simulink model "RM_NSMC"  (R2018b)
settings: Solver=VariableStepAuto  StartTime=0.0  StopTime=100  RelTol=1e-3  EnableMultiTasking=on
settings Model: Creator=Administrator  LastModifiedBy=chengqian
settings OptimizationCC: LifeSpan=inf
settings DebuggingCC: LibraryContextMissingDiagnostic=none  SFUnexpectedBacktrackingDiag=warning  SFNoUnconditionalDefaultTransitionDiag=warning  SFExecutionAtInitializationDiag=none
settings SFSimCC: SimUseLocalCustomCode=off
settings RTWCC: RTWUseLocalCustomCode=off
settings CodeAppCC: StateflowObjectComments=on
settings GRTTargetCC: TargetLangStandard=C89/C90 (ANSI)  GeneratePreprocessorConditionals=Disable all
settings ConfigComp: CovMetricSettings=dw  CovHtmlReporting=on  CovSaveCumulativeToWorkspaceVar=on  CovSaveSingleToWorkspaceVar=on  CovExternalEMLEnable=off

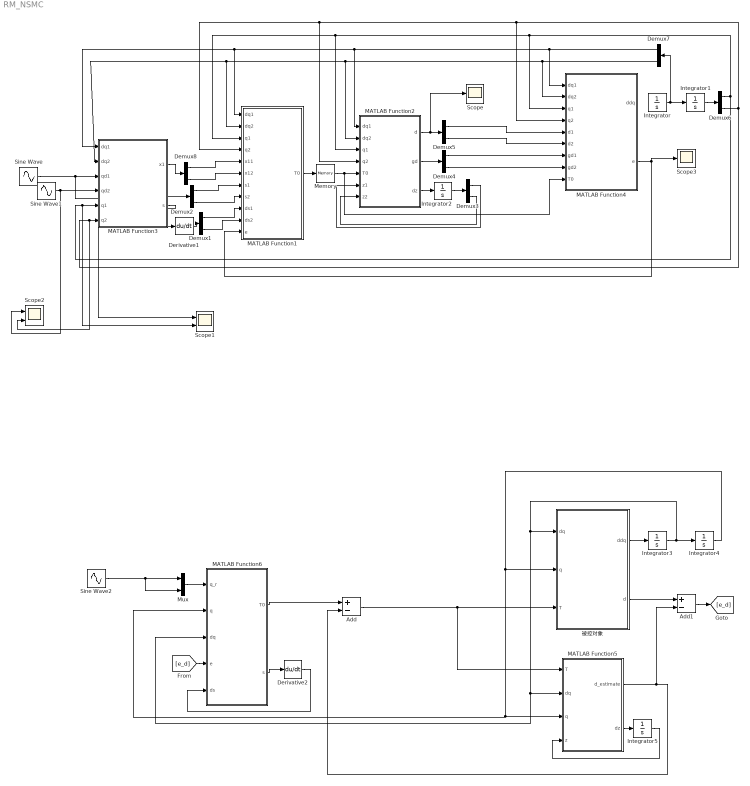
== system RM_NSMC ==
  Add : Sum  Inputs=+-
  Add1 : Sum  Inputs=+-
  Demux{1..8} (8 alike) : Demux  Outputs=2
  Derivative1 : Derivative
  Derivative2 : Derivative
  Integrator{,1..5} (6 alike) : Integrator
  MATLAB Function1 : MATLAB Function  TreatAsAtomicUnit=on
  MATLAB Function2 : MATLAB Function  TreatAsAtomicUnit=on
  MATLAB Function3 : MATLAB Function  TreatAsAtomicUnit=on
  MATLAB Function4 : MATLAB Function  TreatAsAtomicUnit=on
  MATLAB Function5 : MATLAB Function  TreatAsAtomicUnit=on
  MATLAB Function6 : MATLAB Function  TreatAsAtomicUnit=on
  Memory : Memory
  Mux : Mux  Inputs=2
  Scope : Scope
  Scope1 : Scope  NumInputPorts=2
  Scope2 : Scope  NumInputPorts=2
  Scope3 : Scope
  Sine Wave : Sin  SampleTime=0
  Sine Wave1 : Sin  SampleTime=0
  Sine Wave2 : Sin  SampleTime=0
  被控对象 : MATLAB Function  TreatAsAtomicUnit=on
  wires:
  Sine Wave1/1 -> Scope2/1, MATLAB Function3/4(qd2)
  Sine Wave/1 -> Scope1/1, MATLAB Function3/3(qd1)
  ? -> Integrator/1
  Integrator/1 -> Integrator1/1, Demux7/1
  MATLAB Function2/3(dz) -> Integrator2/1
  MATLAB Function3/1(x1) -> Demux8/1
  MATLAB Function3/2(s) -> Derivative1/1, Demux2/1
  Derivative1/1 -> Demux1/1
  Demux1/1 -> MATLAB Function1/9(ds1)
  Demux1/2 -> MATLAB Function1/10(ds2)
  Demux2/1 -> MATLAB Function1/7(s1)
  Demux2/2 -> MATLAB Function1/8(s2)
  Integrator2/1 -> Demux3/1
  Demux3/1 -> MATLAB Function2/6(z1)
  Demux3/2 -> MATLAB Function2/7(z2)
  MATLAB Function2/2(gd) -> Demux4/1
  Demux4/1 -> MATLAB Function4/7(gd1)
  Demux4/2 -> MATLAB Function4/8(gd2)
  MATLAB Function2/1(d) -> Scope/1, Demux5/1
  Demux5/1 -> MATLAB Function4/5(d1)
  Demux5/2 -> MATLAB Function4/6(d2)
  Integrator1/1 -> Demux6/1
  Demux6/1 -> Scope1/2, MATLAB Function3/5(q1), MATLAB Function4/3(q1), MATLAB Function1/3(q1), MATLAB Function2/3(q1)
  Demux7/1 -> MATLAB Function4/1(dq1), MATLAB Function2/1(dq1), MATLAB Function3/1(dq1), MATLAB Function1/1(dq1)
  Demux7/2 -> MATLAB Function4/2(dq2), MATLAB Function2/2(dq2), MATLAB Function3/2(dq2), MATLAB Function1/2(dq2)
  Demux6/2 -> Scope2/2, MATLAB Function3/6(q2), MATLAB Function4/4(q2), MATLAB Function1/4(q2), MATLAB Function2/4(q2)
  MATLAB Function4/2(e) -> Scope3/1, MATLAB Function1/11(e)
  Demux8/1 -> MATLAB Function1/5(x11)
  Demux8/2 -> MATLAB Function1/6(x12)
  MATLAB Function1/1(T0) -> Memory/1
  Memory/1 -> MATLAB Function4/9(T0), MATLAB Function2/5(T0)
  被控对象/1(ddq) -> Integrator3/1
  Integrator3/1 -> 被控对象/1(dq), MATLAB Function6/3(dq), MATLAB Function5/2(dq), Integrator4/1
  Integrator4/1 -> MATLAB Function6/2(q), MATLAB Function5/3(q), 被控对象/2(q)
  Add/1 -> MATLAB Function5/1(T), 被控对象/3(T)
  MATLAB Function5/2(dz) -> Integrator5/1
  Integrator5/1 -> MATLAB Function5/4(z)
  MATLAB Function5/1(d_estimate) -> Add1/2, Add/2
  被控对象/2(d) -> Add1/1
  Add1/1 -> [e_d]
  MATLAB Function6/1(T0) -> Add/1
  MATLAB Function6/2(s) -> Derivative2/1
  Derivative2/1 -> MATLAB Function6/5(ds)
  [e_d] -> MATLAB Function6/4(e)
  Mux/1 -> MATLAB Function6/1(q_r)
  Sine Wave2/1 -> Mux/2, Mux/1

== matlab function RM_NSMC/MATLAB Function1 ==
  data: dq1 input; dq2 input; q1 input; q2 input; x11 input; x12 input; s1 input; T0 output; s2 input; ds1 input; ds2 input; e input
function T0 = fcn(dq1,dq2,q1,q2,x11,x12,s1,s2,ds1,ds2,e)
%#codegen
r = 1;
g = 9.8;
p1 = 0.29;
p2 = 0.076;
p3 = 0.087;
p4 = 0.304;
p5 = 0.087;
s = [s1;s2];
ds = [ds1;ds2];
dq = [dq1;dq2];
x1 = [x11;x12];
M = [p1+p2+2*p3*cos(q2) p2+p3*cos(q2);p2+p3*cos(q2) p2];
M1 = [p1+p2+2*p3*cos(x12) p2+p3*cos(x12);p2+p3*cos(x12) p2];
C = [-p3*dq2*sin(q2) -p3*(dq1+dq2)*sin(q2);p3*dq1*sin(q2) 0];
G = [p4*g*cos(q1)+p5*g*cos(q1+q2);p5*g*cos(q1+q2)];
a = [1;1];
T1 = (C-(2*M)/(3*r))*dq+G-e;
T2 = -M1*a;
T0 = T1+T2;

== matlab function RM_NSMC/MATLAB Function5 ==
  data: T input; dq input; d_estimate output; q input; dz output; z input
function [d_estimate,dz] = fcn(T,dq,q,z)
%#codegen
g = 9.8;
p1 = 0.29;
p2 = 0.076;
p3 = 0.087;
p4 = 0.304;
p5 = 0.087;

L = [1.5 0;0 1.5];
q1 = q(1);
q2 = q(2);
dq1 = dq(1);
dq2 = dq(2);

C = [-p3*dq2*sin(q2) -p3*(dq1+dq2)*sin(q2);p3*dq1*sin(q2) 0];
G = [p4*g*cos(q1)+p5*g*cos(q1+q2);p5*g*cos(q1+q2)];

p = 1.5*[dq1;(dq1+dq2)];
dz = -L*z + L*(C*dq + G - T - p);
d_estimate = z + p;

== matlab function RM_NSMC/MATLAB Function2 ==
  data: dq1 input; d output; dq2 input; q1 input; q2 input; T0 input; z1 input; z2 input; gd output; dz output
function [d,gd,dz] = fcn( dq1,dq2,q1,q2,T0,z1,z2)
%#codegen
g = 9.8;
g = 9.8;
p1 = 0.29;
p2 = 0.076;
p3 = 0.087;
p4 = 0.304;
p5 = 0.087;
L = [1.5 0;0 1.5];
dq = [dq1;dq2];
z = [z1;z2];
sgn = [sign(dq1);sign(dq2)];
C = [-p3*dq2*sin(q2) -p3*(dq1+dq2)*sin(q2);p3*dq1*sin(q2) 0];
G = [p4*g*cos(q1)+p5*g*cos(q1+q2);p5*g*cos(q1+q2)];

d = 0.5*sgn+0.1*dq;

p = 1.5*[dq1;(dq1+dq2)];
gd = z+p;
dz = -L*z+L*(C*dq+G-(T0-gd)-p);

== matlab function RM_NSMC/MATLAB Function3 ==
  data: dq1 input; dq2 input; qd1 input; qd2 input; x1 output; q1 input; q2 input; s output
function [x1,s] = fcn(dq1,dq2,qd1,qd2,q1,q2)
%#codegen
r = 1;
f = 1;
q = [q1;q2];
dq=[dq1;dq2];
qd = [qd1;qd2];
x1 = qd-q;
x2 =-dq;
s =(sign(x1+r*x2)*(sqrt(f*(f+sum(abs(x1+r*x2))))-f)/2)+r*x2;

== matlab function RM_NSMC/MATLAB Function4 ==
  data: dq1 input; dq2 input; q1 input; q2 input; d1 input; d2 input; gd1 input; gd2 input; ddq output; e output; T0 input
function [ddq,e] = fcn(dq1,dq2,q1,q2,d1,d2,gd1,gd2,T0)
%#codegen
g = 9.8;
p1 = 0.29;
p2 = 0.076;
p3 = 0.087;
p4 = 0.304;
p5 = 0.087;
d = [d1;d2];
gd = [gd1;gd2];
dq = [dq1;dq2];
M = [p1+p2+2*p3*cos(q2) p2+p3*cos(q2);p2+p3*cos(q2) p2];
C = [-p3*dq2*sin(q2) -p3*(dq1+dq2)*sin(q2);p3*dq1*sin(q2) 0];
G = [p4*g*cos(q1)+p5*g*cos(q1+q2);p5*g*cos(q1+q2)];
e = d-gd;
ddq = inv(M)*(T0+e-C*dq-G);

== matlab function RM_NSMC/被控对象 ==
  data: dq input; q input; ddq output; T input; d output
function [ddq,d] = fcn(dq,q,T)
%#codegen
g = 9.8;
p1 = 0.29;
p2 = 0.076;
p3 = 0.087;
p4 = 0.304;
p5 = 0.087;

q1 = q(1);
q2 = q(2);

dq1 = dq(1);
dq2 = dq(2);
dq = [dq1;dq2];
M = [p1+p2+2*p3*cos(q2) p2+p3*cos(q2);p2+p3*cos(q2) p2];
C = [-p3*dq2*sin(q2) -p3*(dq1+dq2)*sin(q2);p3*dq1*sin(q2) 0];
G = [p4*g*cos(q1)+p5*g*cos(q1+q2);p5*g*cos(q1+q2)];

d = 0.5*sign(dq)+0.1*dq;%%随机扰动

ddq = inv(M)*(T+d-C*dq-G);

== matlab function RM_NSMC/MATLAB Function6 ==
  data: q_r input; q input; dq input; T0 output; e input; s output; ds input
function [T0,s] = fcn(q_r,q,dq,e,ds)
%#codegen
r = 1;%%哪里是
namuta = 1;
g = 9.8;
p1 = 0.29;
p2 = 0.076;
p3 = 0.087;
p4 = 0.304;
p5 = 0.087;

x1 = q_r - q;
x11 = x1(1);
x12 = x1(2);
x2 = -qd;

q1 = q(1);
q2 = q(2);
dq1 = dq(1);
dq2 = dq(2);
dq = [dq1;dq2];

M = [p1+p2+2*p3*cos(q2) p2+p3*cos(q2);p2+p3*cos(q2) p2];
M1 = [p1+p2+2*p3*cos(x12) p2+p3*cos(x12);p2+p3*cos(x12) p2];
C = [-p3*dq2*sin(q2) -p3*(dq1+dq2)*sin(q2);p3*dq1*sin(q2) 0];
G = [p4*g*cos(q1)+p5*g*cos(q1+q2);p5*g*cos(q1+q2)];

s = sign(x1 + r*x2)*((sqrt(namuta*(namuta + abs(x1 + r*x2)))) - namuta)/2 + r*x2;

A = (ds + sqrt(s)*sign(s))/(ds + sqrt(s));

T_BS = (C-(2*M)/(3*r))*dq+G-e;
T_Vss = -M1*A;
T0 = T_BS + T_Vss;
